simulink model "tp3partie2_v2"  (R2015a)
settings: Solver=ode45  StartTime=0.0  StopTime=2000  RelTol=1e-3
values from neighbouring files (symbols this model uses):
  gama = 1    [tp3partie2.m]
  k = 1    [tp3partie2.m]
  k0 = 2    [tp3partie2.m]
  teta0 = k0/k    (= 2)    [tp3partie2.m]
settings Model: Creator=AMANI  LastModifiedBy=Dano
settings DataIOCC: SaveFormat=StructureWithTime  SignalLoggingSaveFormat=ModelDataLogs
settings HardwareCC: ProdIntDivRoundTo=Zero  ProdEndianess=LittleEndian  ProdHWDeviceType=Specified
settings GRTTargetCC: GeneratePreprocessorConditionals=Use local settings  CombineOutputUpdateFcns=off  GRTInterface=on
settings ConfigComp: CovMetricSettings=dw  CovHtmlReporting=on  CovSaveCumulativeToWorkspaceVar=on  CovSaveSingleToWorkspaceVar=on

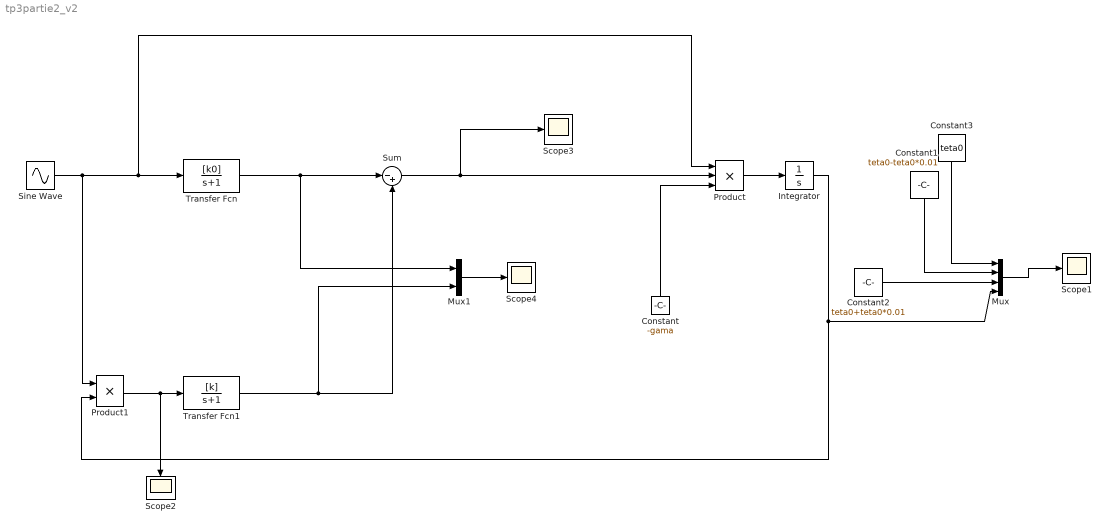
== system tp3partie2_v2 ==
  Constant : Constant  Value=-gama
  Constant1 : Constant  Value=teta0-teta0*0.01
  Constant2 : Constant  Value=teta0+teta0*0.01
  Constant3 : Constant  Value=teta0
  Integrator : Integrator
  Mux : Mux
  Mux1 : Mux  Inputs=2
  Product : Product  Inputs=3
  Product1 : Product
  Scope{1..4} (4 alike) : Scope
      Scope1 settings: YMin=1.701  YMax=2.0335
      Scope3 settings: YMin=-1.86547  YMax=1.73632
      Scope4 settings: YMin=-10  YMax=10  SaveName=ScopeData3
  Sine Wave : Sin  SampleTime=0
  Sum : Sum  Inputs=|-+
  Transfer Fcn : TransferFcn  Numerator=[k0]  Denominator=[1 1]
  Transfer Fcn1 : TransferFcn  Numerator=[k]  Denominator=[1 1]
  wires:
  Transfer Fcn1/1 -> Mux1/2, Sum/2
  Sum/1 -> Scope3/1, Product/2
  Transfer Fcn/1 -> Mux1/1, Sum/1
  Product/1 -> Integrator/1
  Integrator/1 -> Product1/2, Mux/4
  Constant/1 -> Product/3
  Product1/1 -> Scope2/1, Transfer Fcn1/1
  Mux/1 -> Scope1/1
  Constant1/1 -> Mux/2
  Constant2/1 -> Mux/3
  Constant3/1 -> Mux/1
  Sine Wave/1 -> Product1/1, Product/1, Transfer Fcn/1
  Mux1/1 -> Scope4/1
